simulink model "vhz"  (R2023b)
settings: Solver=ode45  StartTime=0  StopTime=1  MaxStep=T_s  RelTol=1e-3  AbsTol=1e-3  EnableMultiTasking=on
values from neighbouring files (symbols this model uses):
  psi_s_ref = 0.95    [init_vhz.m]    (also in task_4_script.m)
  T_L = 14.63    [init_vector.m]    (also in init_vhz.m; task10.m)
  T_s = 125e-6    (= 0.000125)    [init_vector.m]    (also in init_vhz.m; task13_2.m)
libraries: simulink x1
settings Model: Creator=mhinkkan  LastModifiedBy=mikko
settings SolverCC: AutoScaleAbsTol=off  AlgebraicLoopSolver=TrustRegion
settings DataIOCC: SaveFormat=Array  SignalLoggingSaveFormat=ModelDataLogs  SaveOutput=off  SignalLogging=off  DSMLogging=off  SaveTime=off  ReturnWorkspaceOutputs=off
settings OptimizationCC: BlockReduction=off  BooleanDataType=off  DefaultParameterBehavior=Inlined  OptimizeBlockIOStorage=off  BufferReuse=off  ReuseModelBlockBuffer=off  GlobalBufferReuse=off  ExpressionFolding=off  ExpressionDepthLimit=2147483647  LocalBlockOutputs=off  InitFltsAndDblsToZero=on  LifeSpan=inf
settings DebuggingCC: SaveWithParameterizedLinksMsg=none  UnderspecifiedInitializationDetection=Classic  MergeDetectMultiDrivingBlocksExec=none  SignalResolutionControl=TryResolveAllWithWarning  MultiTaskDSMMsg=warning  MultiTaskCondExecSysMsg=none  FcnCallInpInsideContextMsg=warning  UnconnectedInputMsg=warning  UnconnectedOutputMsg=warning  UnconnectedLineMsg=warning  StateNameClashWarn=warning  SFUnexpectedBacktrackingDiag=warning  SFNoUnconditionalDefaultTransitionDiag=warning  ArithmeticOperatorsInVariantConditions=warning
settings HardwareCC: ProdBitPerPointer=32  ProdBitPerSizeT=32  ProdBitPerPtrDiffT=32  ProdLargestAtomicFloat=None  ProdIntDivRoundTo=Undefined  ProdEndianess=Unspecified  ProdWordSize=32  ProdHWDeviceType=32-bit Generic  TargetUnknown=on
settings ModelReferenceCC: EnableRefExpFcnMdlSchedulingChecks=on  PropagateSignalLabelsOutOfModel=off
settings SFSimCC: SimUseLocalCustomCode=off  CustomCodeUndefinedFunction=UseInterfaceOnly
settings RTWCC: RTWUseLocalCustomCode=off
settings CodeAppCC: StateflowObjectComments=on
settings GRTTargetCC: TargetFcnLib=ansi_tfl_tmw.mat  TargetLangStandard=C89/C90 (ANSI)  CombineOutputUpdateFcns=off  GRTInterface=on
settings ConfigComp: CovMetricSettings=dw  CovSaveCumulativeToWorkspaceVar=on  CovSaveSingleToWorkspaceVar=on  CovExternalEMLEnable=off

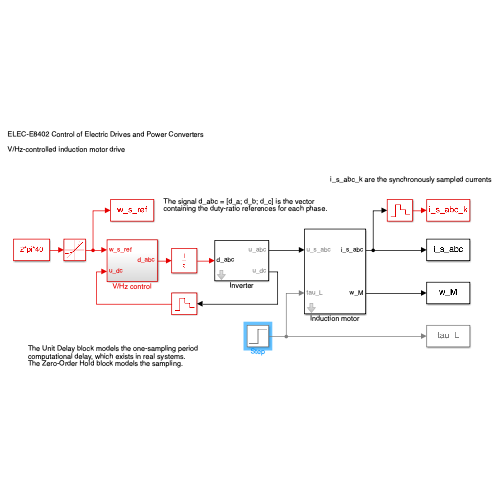
[thumbnail: Simulink's stored preview of the top-level diagram]
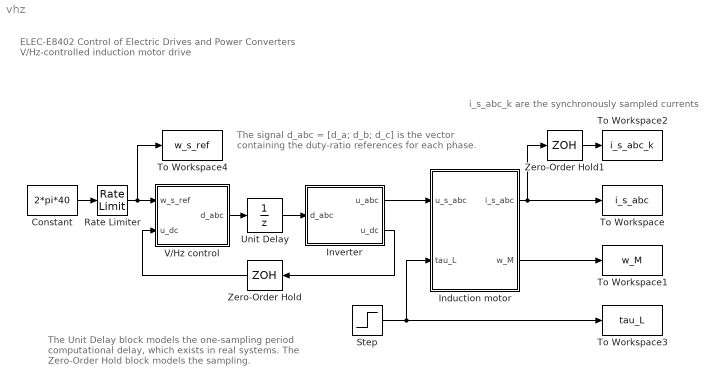
== system vhz ==
  note: i_s_abc_k are the synchronously sampled currents
  note: The signal d_abc = [d_a; d_b; d_c] is the vector
      | containing the duty-ratio references for each phase.
  note: ELEC-E8402 Control of Electric Drives and Power Converters
      |
      | V/Hz-controlled induction motor drive
  note: The Unit Delay block models the one-sampling period
      | computational delay, which exists in real systems.
      | The Zero-Order Hold block models the sampling.
  Constant : Constant  Value=2*pi*40  SampleTime=T_s
  Induction motor : Subsystem  mask{R_s=3.7, R_R=2.1, L_sigma=0.021, L_M=0.224, n_p=2, J=0.015}
      mask prompts: R_s "Stator resistance R_s (ohm)"; R_R "Rotor resistance R_R (ohm)"; L_sigma "Leakage inductance L_sigma (H)"; L_M "Magnetizing inductance L_M (H)"; n_p "Number of pole pairs n_p"; J "Total inertia J (kgm^2)"
      mask help: Inverse-Gamma model
  Inverter : Subsystem  mask{T_s=T_s, u_dc=540}
      mask prompts: T_s "Sampling period T_s (s)"; u_dc "DC-link voltage u_dc (V)"
      mask help: The switching period is 2*Ts and the switching frequency is 1/(2*Ts).
  Rate Limiter : RateLimiter  RisingSlewLimit=2*pi*100  FallingSlewLimit=-2*pi*100  SampleTimeMode=inherited
  Step : Step  Time=.6  After=T_L  SampleTime=0
  To Workspace : ToWorkspace  VariableName=i_s_abc  SaveFormat=Timeseries  SampleTime=-1
  To Workspace1 : ToWorkspace  VariableName=w_M  SaveFormat=Timeseries  SampleTime=-1
  To Workspace2 : ToWorkspace  VariableName=i_s_abc_k  SaveFormat=Timeseries  SampleTime=-1
  To Workspace3 : ToWorkspace  VariableName=tau_L  SaveFormat=Timeseries  SampleTime=-1
  To Workspace4 : ToWorkspace  VariableName=w_s_ref  SaveFormat=Timeseries  SampleTime=-1
  Unit Delay : UnitDelay  SampleTime=T_s  HasFrameUpgradeWarning=on
  V/Hz control : Subsystem
  Zero-Order Hold : ZeroOrderHold  SampleTime=T_s
  Zero-Order Hold1 : ZeroOrderHold  SampleTime=T_s
  wires:
  Step/1 -> Induction motor/2(tau_L), To Workspace3/1
  Inverter/1(u_abc) -> Induction motor/1(u_s_abc)
  Induction motor/1(i_s_abc) -> Zero-Order Hold1/1, To Workspace/1
  Induction motor/2(w_M) -> To Workspace1/1
  Unit Delay/1 -> Inverter/1(d_abc)
  Zero-Order Hold/1 -> V/Hz control/2(u_dc)
  V/Hz control/1(d_abc) -> Unit Delay/1
  Constant/1 -> Rate Limiter/1
  Rate Limiter/1 -> To Workspace4/1, V/Hz control/1(w_s_ref)
  Inverter/2(u_dc) -> Zero-Order Hold/1
  Zero-Order Hold1/1 -> To Workspace2/1

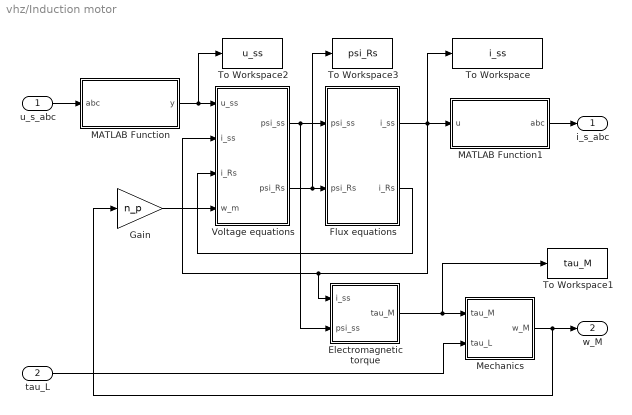
== system vhz/Induction motor ==
  u_s_abc : Inport
  tau_L : Inport  Port=2
  Electromagnetic torque : Subsystem
  Flux equations : Subsystem
  Gain : Gain  Gain=n_p  SaturateOnIntegerOverflow=on  OutDataTypeStr=Inherit: Same as input  ParamDataTypeStr=Inherit: Same as input
  MATLAB Function : MATLAB Function  TreatAsAtomicUnit=on
  MATLAB Function1 : MATLAB Function  TreatAsAtomicUnit=on
  Mechanics : Subsystem
  To Workspace : ToWorkspace  VariableName=i_ss  SaveFormat=Timeseries  SampleTime=-1
  To Workspace1 : ToWorkspace  VariableName=tau_M  SaveFormat=Timeseries  SampleTime=-1
  To Workspace2 : ToWorkspace  VariableName=u_ss  SaveFormat=Timeseries  SampleTime=-1
  To Workspace3 : ToWorkspace  VariableName=psi_Rs  SaveFormat=Timeseries  SampleTime=-1
  Voltage equations : Subsystem
  i_s_abc : Outport
  w_M : Outport  Port=2
  wires:
  tau_L/1 -> Mechanics/2(tau_L)
  Mechanics/1(w_M) -> w_M/1, Gain/1
  Flux equations/1(i_ss) -> To Workspace/1, MATLAB Function1/1(u), Voltage equations/2(i_ss), Electromagnetic torque/1(i_ss)
  u_s_abc/1 -> MATLAB Function/1(abc)
  Voltage equations/2(psi_Rs) -> To Workspace3/1, Flux equations/2(psi_Rs)
  Voltage equations/1(psi_ss) -> Electromagnetic torque/2(psi_ss), Flux equations/1(psi_ss)
  Flux equations/2(i_Rs) -> Voltage equations/3(i_Rs)
  Electromagnetic torque/1(tau_M) -> To Workspace1/1, Mechanics/1(tau_M)
  MATLAB Function/1(y) -> To Workspace2/1, Voltage equations/1(u_ss)
  MATLAB Function1/1(abc) -> i_s_abc/1
  Gain/1 -> Voltage equations/4(w_m)

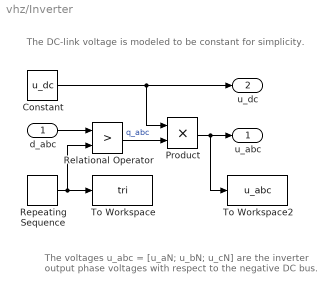
== system vhz/Inverter ==
  note: The voltages u_abc = [u_aN; u_bN; u_cN] are the inverter
      | output phase voltages with respect to the negative DC bus.
  note: The DC-link voltage is modeled to be constant for simplicity.
  d_abc : Inport
  Constant : Constant  Value=u_dc  SampleTime=0
  Product : Product
  Relational Operator : RelationalOperator  Operator=>  OutDataTypeStr=boolean  InputSameDT=off
  Repeating Sequence : simulink/Sources/Repeating Sequence  rep_seq_t=[0 1 2]*T_s  rep_seq_y=[1 0 1]
  To Workspace : ToWorkspace  VariableName=tri  SaveFormat=Timeseries  SampleTime=-1
  To Workspace2 : ToWorkspace  VariableName=u_abc  SaveFormat=Timeseries  SampleTime=-1
  u_abc : Outport
  u_dc : Outport  Port=2
  wires:
  Repeating Sequence/1 -> Relational Operator/2, To Workspace/1
  d_abc/1 -> Relational Operator/1
  Relational Operator/1 -> Product/2  "q_abc"
  Constant/1 -> Product/1, u_dc/1
  Product/1 -> u_abc/1, To Workspace2/1

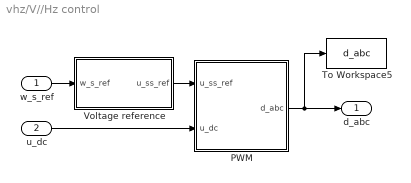
== system vhz/V//Hz control ==
  w_s_ref : Inport
  u_dc : Inport  Port=2
  PWM : Subsystem
  To Workspace5 : ToWorkspace  VariableName=d_abc  SaveFormat=Timeseries  SampleTime=-1
  Voltage reference : Subsystem
  d_abc : Outport
  wires:
  w_s_ref/1 -> Voltage reference/1(w_s_ref)
  Voltage reference/1(u_ss_ref) -> PWM/1(u_ss_ref)
  u_dc/1 -> PWM/2(u_dc)
  PWM/1(d_abc) -> d_abc/1, To Workspace5/1

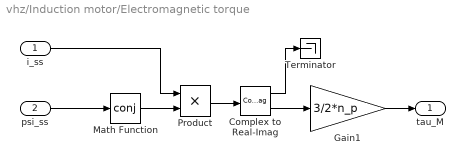
== system vhz/Induction motor/Electromagnetic torque ==
  i_ss : Inport
  psi_ss : Inport  Port=2
  Complex to Real-Imag : ComplexToRealImag
  Gain1 : Gain  Gain=3/2*n_p
  Math Function : Math  Operator=conj
  Product : Product
  Terminator : Terminator
  tau_M : Outport
  wires:
  i_ss/1 -> Product/1
  Math Function/1 -> Product/2
  Product/1 -> Complex to Real-Imag/1
  Complex to Real-Imag/2 -> Gain1/1
  Gain1/1 -> tau_M/1
  psi_ss/1 -> Math Function/1
  Complex to Real-Imag/1 -> Terminator/1

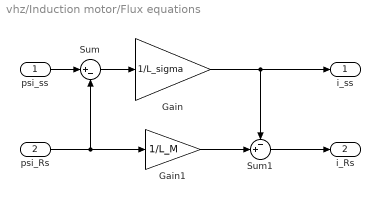
== system vhz/Induction motor/Flux equations ==
  psi_ss : Inport
  psi_Rs : Inport  Port=2
  Gain : Gain  Gain=1/L_sigma
  Gain1 : Gain  Gain=1/L_M
  Sum : Sum  Inputs=|+-
  Sum1 : Sum  Inputs=-+|
  i_ss : Outport
  i_Rs : Outport  Port=2
  wires:
  psi_Rs/1 -> Gain1/1, Sum/2
  Gain1/1 -> Sum1/2
  Sum1/1 -> i_Rs/1
  psi_ss/1 -> Sum/1
  Sum/1 -> Gain/1
  Gain/1 -> Sum1/1, i_ss/1

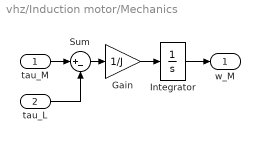
== system vhz/Induction motor/Mechanics ==
  tau_M : Inport
  tau_L : Inport  Port=2
  Gain : Gain  Gain=1/J  SaturateOnIntegerOverflow=on  OutDataTypeStr=Inherit: Same as input  ParamDataTypeStr=Inherit: Same as input
  Integrator : Integrator
  Sum : Sum  Inputs=|+-  InputSameDT=on  SaturateOnIntegerOverflow=on  OutDataTypeStr=Inherit: Same as first input
  w_M : Outport
  wires:
  tau_L/1 -> Sum/2
  Sum/1 -> Gain/1
  Gain/1 -> Integrator/1
  Integrator/1 -> w_M/1
  tau_M/1 -> Sum/1

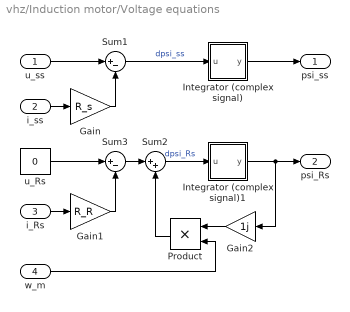
== system vhz/Induction motor/Voltage equations ==
  u_ss : Inport
  i_ss : Inport  Port=2
  i_Rs : Inport  Port=3
  w_m : Inport  Port=4
  Gain : Gain  Gain=R_s
  Gain1 : Gain  Gain=R_R
  Gain2 : Gain  Gain=1j
  Integrator (complex signal) : Subsystem
      mask Display: disp('1/s');
  Integrator (complex signal)1 : Subsystem
      mask Display: disp('1/s');
  Product : Product  RndMeth=Zero
  Sum1 : Sum  Inputs=|+-
  Sum2 : Sum  Inputs=|++
  Sum3 : Sum  Inputs=|+-
  u_Rs : Constant  Value=0  SampleTime=0
  psi_ss : Outport
  psi_Rs : Outport  Port=2
  wires:
  u_ss/1 -> Sum1/1
  i_ss/1 -> Gain/1
  Sum1/1 -> Integrator (complex signal)/1(u)  "dpsi_ss"
  Gain/1 -> Sum1/2
  Integrator (complex signal)/1(y) -> psi_ss/1
  u_Rs/1 -> Sum3/1
  i_Rs/1 -> Gain1/1
  Gain1/1 -> Sum3/2
  Sum3/1 -> Sum2/1
  Sum2/1 -> Integrator (complex signal)1/1(u)  "dpsi_Rs"
  Product/1 -> Sum2/2
  Integrator (complex signal)1/1(y) -> psi_Rs/1, Gain2/1
  Gain2/1 -> Product/1
  w_m/1 -> Product/2

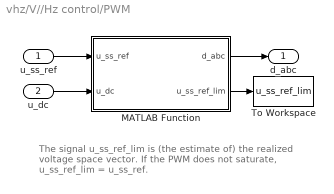
== system vhz/V//Hz control/PWM ==
  note: The signal u_ss_ref_lim is (the estimate of) the realized
      | voltage space vector. If the PWM does not
      | saturate, u_ss_ref_lim = u_ss_ref.
  u_ss_ref : Inport
  u_dc : Inport  Port=2
  MATLAB Function : MATLAB Function  TreatAsAtomicUnit=on
  To Workspace : ToWorkspace  VariableName=u_ss_ref_lim  SaveFormat=Timeseries  SampleTime=-1
  d_abc : Outport
  wires:
  u_ss_ref/1 -> MATLAB Function/1(u_ss_ref)
  u_dc/1 -> MATLAB Function/2(u_dc)
  MATLAB Function/1(d_abc) -> d_abc/1
  MATLAB Function/2(u_ss_ref_lim) -> To Workspace/1

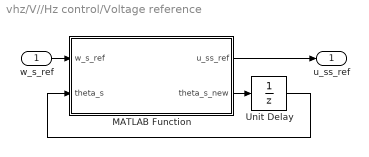
== system vhz/V//Hz control/Voltage reference ==
  w_s_ref : Inport
  MATLAB Function : MATLAB Function  TreatAsAtomicUnit=on
  Unit Delay : UnitDelay  SampleTime=-1  HasFrameUpgradeWarning=on
  u_ss_ref : Outport
  wires:
  Unit Delay/1 -> MATLAB Function/2(theta_s)
  w_s_ref/1 -> MATLAB Function/1(w_s_ref)
  MATLAB Function/1(u_ss_ref) -> u_ss_ref/1
  MATLAB Function/2(theta_s_new) -> Unit Delay/1

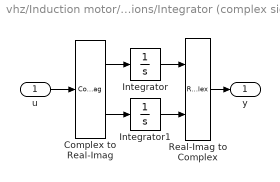
== system vhz/Induction motor/Voltage equations/Integrator (complex signal) ==
  u : Inport
  Complex to Real-Imag : ComplexToRealImag
  Integrator : Integrator
  Integrator1 : Integrator
  Real-Imag to Complex : RealImagToComplex
  y : Outport
  wires:
  Complex to Real-Imag/1 -> Integrator/1
  Complex to Real-Imag/2 -> Integrator1/1
  Integrator/1 -> Real-Imag to Complex/1
  Integrator1/1 -> Real-Imag to Complex/2
  Real-Imag to Complex/1 -> y/1
  u/1 -> Complex to Real-Imag/1

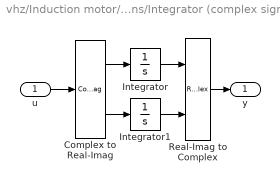
== system vhz/Induction motor/Voltage equations/Integrator (complex signal)1 ==
  u : Inport
  Complex to Real-Imag : ComplexToRealImag
  Integrator : Integrator
  Integrator1 : Integrator
  Real-Imag to Complex : RealImagToComplex
  y : Outport
  wires:
  Complex to Real-Imag/1 -> Integrator/1
  Complex to Real-Imag/2 -> Integrator1/1
  Integrator/1 -> Real-Imag to Complex/1
  Integrator1/1 -> Real-Imag to Complex/2
  Real-Imag to Complex/1 -> y/1
  u/1 -> Complex to Real-Imag/1

== matlab function vhz/V//Hz control/PWM/MATLAB Function ==
  data: u_ss_ref input; u_dc input; d_abc output; u_ss_ref_lim output
function [d_abc, u_ss_ref_lim] = pwm(u_ss_ref, u_dc)

% Components of the voltage space vector
u_alpha_ref = real(u_ss_ref);
u_beta_ref  = imag(u_ss_ref);

% Phase-voltage references
u_a_ref = u_alpha_ref;
u_b_ref = .5*(-u_alpha_ref + sqrt(3)*u_beta_ref);
u_c_ref = .5*(-u_alpha_ref - sqrt(3)*u_beta_ref);

% Vector of phase-voltage references
u_abc_ref = [u_a_ref; u_b_ref; u_c_ref];

% Symmetrization of the references by adding the zero-sequence voltage
u0 = .5*(max(u_abc_ref) + min(u_abc_ref));
u_abc_ref = u_abc_ref - u0;

% Clamping of the reference voltages such that no phase error is caused. 
% If all phase voltage reference are realizable (below Udc/2), m = 1 holds.
m = max([2*u_abc_ref/u_dc; 1]);
u_abc_ref = u_abc_ref/m;

% Duty cycles, which can be directly used for triangle comparison, 
% if the triangle wave varies between 0...1
d_abc = .5 + u_abc_ref/u_dc;

% Realized voltage vector is calculated from the clamped duty ratios.
% If the PWM does not saturate, u_ss_ref_lim = u_ss_ref holds. The realized
% voltage vector is needed, e.g., for the current-controller antiwindup.
u_ss_ref_lim = 2/3*(d_abc(1) + d_abc(2)*exp(1j*2*pi/3) ...
    + d_abc(3)*exp(1j*4*pi/3))*u_dc;

== matlab function vhz/V//Hz control/Voltage reference/MATLAB Function ==
  data: u_ss_ref output size=1; w_s_ref input size=1; theta_s input size=1; psi_s_ref parameter size=1; theta_s_new output size=1; T_s parameter size=1
function [u_ss_ref, theta_s_new] = vhz(w_s_ref, theta_s, psi_s_ref, T_s)

% Voltage vector
% Note: 1j is the imaginary unit in MATLAB
% u_ss_ref = ...  % Complete this
u_ss_ref = psi_s_ref*w_s_ref*exp(1j*theta_s);

% Update (integrate) the voltage angle
theta_s_new = theta_s + T_s*w_s_ref;

% Extra information about MATLAB Functions: 
% The inputs, ouputs, and parameters of MATLAB Functions can be defined by 
% clicking the "Edit Data" button in the toolstrip above. For example, T_s
% and psi_s_ref are defined to be parameters, which means that their values
% are read from the workspace. In this assignment, you don't need to change
% these settings.

== matlab function vhz/Induction motor/MATLAB Function1 ==
  data: u input size=1; abc output size=3
function abc = alphabeta2abc(u)

a = real(u);
b = real(exp(1j*4*pi/3)*u);
c = real(exp(1j*2*pi/3)*u);

abc = [a; b; c];

== matlab function vhz/Induction motor/MATLAB Function ==
  data: abc input size=3; y output size=1
function y = abc2alphabeta(abc)

y = 2/3*(abc(1) + exp(1j*2*pi/3)*abc(2) + exp(1j*4*pi/3)*abc(3));
